simulink model "DynamicSimulinkModel"  (R2024a)
settings: Solver=VariableStepAuto  StartTime=0.0  StopTime=100  RelTol=1e-3
undefined symbols (not defined in the file): OCV, R0
settings Model: Creator=vboutrou  LastModifiedBy=vboutrou

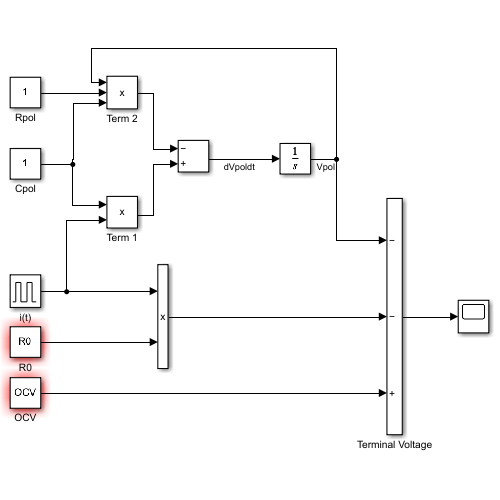
[thumbnail: Simulink's stored preview of the top-level diagram]
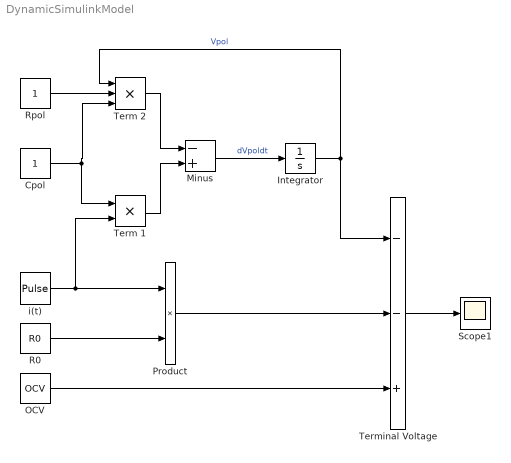
== system DynamicSimulinkModel ==
  Cpol : Constant
  Integrator : Integrator
  Minus : Sum  Inputs=-+
  OCV : Constant  Value=OCV
  Product : Product
  R0 : Constant  Value=R0
  Rpol : Constant
  Scope1 : Scope
  Term 1 : Product  Inputs=**
  Term 2 : Product  Inputs=***
  Terminal Voltage : Sum  Inputs=--+
  i(t) : DiscretePulseGenerator  PulseType=Time based  Period=10  PulseWidth=30  PhaseDelay=2
  wires:
  Minus/1 -> Integrator/1  "dVpoldt"
  Integrator/1 -> Term 2/1, Terminal Voltage/1  "Vpol"
  Rpol/1 -> Term 2/2
  Cpol/1 -> Term 2/3, Term 1/1
  i(t)/1 -> Term 1/2, Product/1
  Term 2/1 -> Minus/1
  Term 1/1 -> Minus/2
  R0/1 -> Product/2
  Terminal Voltage/1 -> Scope1/1
  OCV/1 -> Terminal Voltage/3
  Product/1 -> Terminal Voltage/2
